simulink model "verify_com_acceleration_computation"  (R2015a)
settings: Solver=ode45  StartTime=0.0  StopTime=1.2  RelTol=1e-3
undefined symbols (not defined in the file or in its folder): A_kalman_transverse, A_kalman_vertical, B_kalman_transverse, B_kalman_vertical, C_kalman_transverse, C_kalman_vertical, com_leg_motor, com_torso, Discrete, g, initial_dx_estimate, initial_dy_estimate, initial_dz_estimate, initial_z_estimate, kalman_stance_slip_threshold, lateral_offset, m_leg, m_leg_motor, m_torso, m_total_real, P0_kalman_transverse, P0_kalman_vertical, pelvis_to_imu, R_kalman_accelerometer, R_kalman_foot_slip, R_kalman_foot_stance, sample_time, Time, X, Y, Z
libraries: nesl_utility x121, sm_lib x43, simulink x3, ctrlSharedLib x3
(part 1 of 3)
settings Model: Creator=wmartin  LastModifiedBy=wmartin

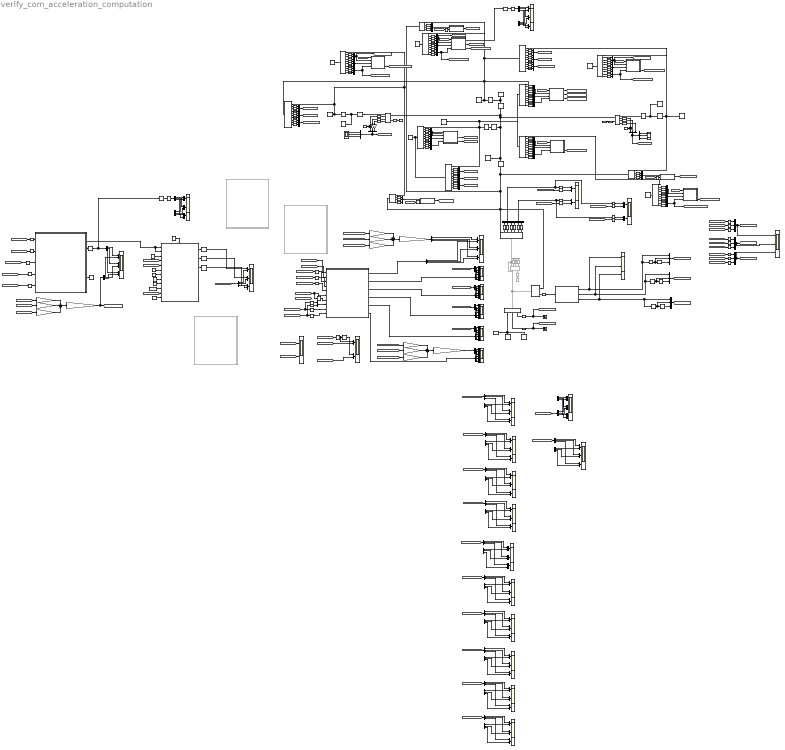
== system verify_com_acceleration_computation ==
  COM Acceleration Yawed Frame : Scope  NumInputPorts=3
      settings: YMin=-0.7~-1.75~-25  YMax=0.7~1.75~5  SaveName=ScopeData29  SampleInput=on
  COM from pelvis : Scope  NumInputPorts=3
      settings: YMin=-0.125~-0.175~-0.15  YMax=0.125~0.2~0.125  SaveName=ScopeData12  SampleInput=on
  Cartesian Joint : sm_lib/Joints/Cartesian Joint  SenseConstraintForce=off  SenseConstraintForceX=off  SenseConstraintForceY=off  SenseConstraintForceZ=off  SenseConstraintTorque=off  SenseConstraintTorqueX=off  SenseConstraintTorqueY=off  SenseConstraintTorqueZ=off  SenseTotalForce=off  SenseTotalForceX=off  SenseTotalForceY=off  SenseTotalForceZ=off  SenseTotalTorque=off  SenseTotalTorqueX=off  SenseTotalTorqueY=off  SenseTotalTorqueZ=off  CompositeWrenchDir=FollowerOnBase  CompositeWrenchFrame=BaseFrame  PxEquilibriumPosition=0  PxEquilibriumPositionUnits=m  PxSpringStiffness=0  PxSpringStiffnessUnits=N/m  PxDampingCoefficient=0  PxDampingCoefficientUnits=N/(m/s)  PxTorqueActuationMode=NoTorque  PxMotionActuationMode=ComputedMotion  PxSensePosition=off  PxSenseVelocity=off  PxSenseAcceleration=off  PxSenseTorqueForce=off  PxPositionTargetSpecify=off  PxPositionTargetPriority=High  PxPositionTargetValue=0  PxPositionTargetValueUnits=m  PxVelocityTargetSpecify=off  PxVelocityTargetPriority=High  PxVelocityTargetValue=0  PxVelocityTargetValueUnits=m/s  PyEquilibriumPosition=0  PyEquilibriumPositionUnits=m  PySpringStiffness=0  PySpringStiffnessUnits=N/m  PyDampingCoefficient=0  PyDampingCoefficientUnits=N/(m/s)  PyTorqueActuationMode=InputTorque  PyMotionActuationMode=ComputedMotion  PySensePosition=off  PySenseVelocity=off  PySenseAcceleration=off  PySenseTorqueForce=off  PyPositionTargetSpecify=off  PyPositionTargetPriority=High  PyPositionTargetValue=0  PyPositionTargetValueUnits=m  PyVelocityTargetSpecify=off  PyVelocityTargetPriority=High  PyVelocityTargetValue=0  PyVelocityTargetValueUnits=m/s  PzEquilibriumPosition=0  PzEquilibriumPositionUnits=m  PzSpringStiffness=0  PzSpringStiffnessUnits=N/m  PzDampingCoefficient=0  PzDampingCoefficientUnits=N/(m/s)  PzTorqueActuationMode=InputTorque  PzMotionActuationMode=ComputedMotion  PzSensePosition=off  PzSenseVelocity=off  PzSenseAcceleration=off  PzSenseTorqueForce=off  PzPositionTargetSpecify=off  PzPositionTargetPriority=High  PzPositionTargetValue=0  PzPositionTargetValueUnits=m  PzVelocityTargetSpecify=off  PzVelocityTargetPriority=High  PzVelocityTargetValue=0  PzVelocityTargetValueUnits=m/s  BlockFunction=simmechanics.library.joints.cartesian_joint
  Compute COM Translational Acceleration (IMU uses non-rotating measurement frame) : MATLAB Function  TreatAsAtomicUnit=on
  Compute COM Translational Acceleration (IMU uses non-rotating measurement frame) (yawed frame as rotated world frame - non rotating) : MATLAB Function  Commented=on  TreatAsAtomicUnit=on
  Compute COM Translational Acceleration (IMU uses rotating measurement frame)1 : MATLAB Function  Commented=on  TreatAsAtomicUnit=on
  Compute COM Translational Acceleration (IMU uses non-rotating measurement frame) : MATLAB Function  Commented=on  TreatAsAtomicUnit=on
  Constant{,1..2,11} (4 alike) : Constant  Value=0
  Constant10 : Constant  Value=true
  Constant12 : Constant  Value=false
  Constant3 : Constant  Value=pi/2
  Constant4 : Constant  Value=pi/2
  Constant5 : Constant  Commented=on  Value=0
  Constant6 : Constant  Value=1000
  Constant7 : Constant  Value=[0 0 0]
  Constant8 : Constant  Value=[0 0 0]
  Constant9 : Constant  Value=[0.1 0 0]
  Demux{,1..42,44..45} (45 alike) : Demux  Outputs=3
  Derivative{,1..12} (13 alike) : Derivative
  Gain{,1,6..7,10..11} (6 alike) : Gain  Gain=m_leg_motor+m_leg
  Gain12 : Gain  Gain=m_torso
  Gain13 : Gain  Gain=1/(m_torso+2*(m_leg_motor+m_leg))
  Gain2 : Gain  Gain=m_torso
  Gain3 : Gain  Gain=1/(m_torso+2*(m_leg_motor+m_leg))
  Gain4 : Gain  Gain=-1
  Gain5 : Gain  Gain=-1
  Gain8 : Gain  Gain=m_torso
  Gain9 : Gain  Gain=1/(m_torso+2*(m_leg_motor+m_leg))
  IMU : sm_lib/Body Elements/Graphic  GraphicType=Marker  MarkerShape=Sphere  MarkerSize=10  MarkerSizeUnits=m  GraphicVisPropType=SimpleVisualProperties  GraphicDiffuseColor=[0.0 0.8 0.8]  GraphicSpecularColor=[0.5 0.5 0.5 1.0]  GraphicAmbientColor=[0.15 0.15 0.15 1.0]  GraphicEmissiveColor=[0.0 0.0 0.0 1.0]  GraphicShininess=75  GraphicOpacity=1.0  BlockFunction=simmechanics.library.body_elements.graphic
  IMU Acceleration Yawed : Scope  NumInputPorts=3
      settings: YMin=-0.3~-1.5~-10  YMax=0.45~6~7  SaveName=ScopeData9  SampleInput=on
  IMU Velocity Yawed : Scope  NumInputPorts=3
      settings: YMin=-0.45~-0.25~-15  YMax=0.2~4~1  SaveName=ScopeData11  SampleInput=on
  Imu to Torso COM yawed : Scope  NumInputPorts=3
      settings: YMin=-0.1175~0.12~-0.2  YMax=-0.095~0.23~0.15  SaveName=ScopeData10  SampleInput=on
  Kalman Filter : Scope  NumInputPorts=3
      settings: YMin=-1000~-1500~-25  YMax=1500~750~35  SaveName=ScopeData23  SampleInput=on
  Kalman Filtering : Subsystem
  L Hip Graphic : sm_lib/Body Elements/Graphic  GraphicType=Marker  MarkerShape=Sphere  MarkerSize=10  MarkerSizeUnits=m  GraphicVisPropType=SimpleVisualProperties  GraphicDiffuseColor=[0.0 0.2 1.0]  GraphicSpecularColor=[0.5 0.5 0.5 1.0]  GraphicAmbientColor=[0.15 0.15 0.15 1.0]  GraphicEmissiveColor=[0.0 0.0 0.0 1.0]  GraphicShininess=75  GraphicOpacity=1.0  BlockFunction=simmechanics.library.body_elements.graphic
  L Hip Yawed : Scope  NumInputPorts=3
      settings: YMin=0.95~0.95~-5  YMax=1.05~1.05~5  SaveName=ScopeData8  SampleInput=on
  LHip  body frame : Scope  NumInputPorts=3
      settings: YMin=0.95~0.95~-5  YMax=1.05~1.05~5  SaveName=ScopeData21  SampleInput=on
  Left Hip Acceleration World Frame : Scope  NumInputPorts=3
      settings: YMin=-0.3~-10~-27.5  YMax=0.9~12.5~7.5  SaveName=ScopeData28  SampleInput=on
  Left Hip Angular Positions / Velocities / Accelerations : Scope  NumInputPorts=3
      settings: YMin=0.95~0.95~-5  YMax=1.05~1.05~5  SaveName=ScopeData2  SampleInput=on
  Left Hip Joint : sm_lib/Joints/Revolute Joint  SenseConstraintForce=off  SenseConstraintForceX=off  SenseConstraintForceY=off  SenseConstraintForceZ=off  SenseConstraintTorque=off  SenseConstraintTorqueX=off  SenseConstraintTorqueY=off  SenseConstraintTorqueZ=off  SenseTotalForce=off  SenseTotalForceX=off  SenseTotalForceY=off  SenseTotalForceZ=off  SenseTotalTorque=off  SenseTotalTorqueX=off  SenseTotalTorqueY=off  SenseTotalTorqueZ=off  CompositeWrenchDir=FollowerOnBase  CompositeWrenchFrame=BaseFrame  EquilibriumPosition=0  EquilibriumPositionUnits=deg  SpringStiffness=0  SpringStiffnessUnits=N*m/deg  DampingCoefficient=0  DampingCoefficientUnits=N*m/(deg/s)  TorqueActuationMode=InputTorque  MotionActuationMode=ComputedMotion  SensePosition=on  SenseVelocity=on  SenseAcceleration=on  SenseTorqueForce=off  PositionTargetSpecify=off  PositionTargetPriority=High  PositionTargetValue=0  PositionTargetValueUnits=deg  VelocityTargetSpecify=off  VelocityTargetPriority=High  VelocityTargetValue=0  VelocityTargetValueUnits=deg/s  BlockFunction=simmechanics.library.joints.revolute_joint
  Left Hip Mass : sm_lib/Body Elements/Solid  InertiaType=Custom  Mass=m_leg_motor+m_leg  MassUnits=kg  CenterOfMass=com_leg_motor  CenterOfMassUnits=m  MomentsOfInertia=[1 1 1]  MomentsOfInertiaUnits=kg*m^2  ProductsOfInertia=[0 0 0]  ProductsOfInertiaUnits=kg*m^2  DensityBased=on  Density=1000  DensityUnits=kg/(m^3)  GraphicType=None  MarkerShape=Sphere  MarkerSize=10  MarkerSizeUnits=m  GraphicVisPropType=SimpleVisualProperties  GraphicDiffuseColor=[0.5 0.5 0.5]  GraphicSpecularColor=[0.5 0.5 0.5 1.0]  GraphicAmbientColor=[0.15 0.15 0.15 1.0]  GraphicEmissiveColor=[0.0 0.0 0.0 1.0]  GraphicShininess=75  GraphicOpacity=1.0  GeometryShape=Sphere  RectangleSize=[1 1]  RectangleSizeUnits=m  BrickDimensions=[1 1 1]  BrickDimensionUnits=m  CylinderRadius=1  CylinderRadiusUnits=m  CylinderLength=1  CylinderLengthUnits=m  SphereRadius=0.15  SphereRadiusUnits=m  EllipsoidRadii=[1 1 1]  EllipsoidRadiiUnits=m  ExtrusionCrossSection=[1 1; -1 1; -1 -1; 1 -1]  ExtrusionCrossSectionUnits=m  ExtrusionLength=1  ExtrusionLengthUnits=m  PolygonNumSides=3  PolygonOuterRadius=1  PolygonOuterRadiusUnits=m  ExtGeomFileType=STL  ExtGeomFileUnits=m  RevolutionCrossSection=[1 1; 1 -1; 2 -1; 2 1]  RevolutionCrossSectionUnits=m  RevolutionExtent=Full  RevolutionAngle=180  RevolutionAngleUnits=deg  BlockFunction=simmechanics.library.body_elements.solid
  Mechanism Configuration : sm_lib/Utilities/Mechanism Configuration  UniformGravity=Constant  GravityVector=[0 0 -9.80665]  GravityUnits=m/s^2  LinearizationDelta=0.001  BlockFunction=simmechanics.library.utilities.mechanism_configuration
  Mux{1..4,10..12,26..27,32..36,38,45..50,52,57,61..63,67..68,73..81,85..87,91..93} (43 alike) : Mux  Inputs=3
  Mux{5..9,13..25,28..31,37,39..41,43..44,51,53..56,58..60,64..66,69..72,82..84,88..90,94..117} (73 alike) : Mux  Inputs=2
  Mux42 : Mux  Commented=on  Inputs=3
  PS-Simulink Converter{,1..42,46..114} (112 alike) : nesl_utility/PS-Simulink Converter  PhysicalDomain=network_engine_domain  SubClassName=ps_output  LeftPortType=input  RightPortType=output  PseudoPeriodic=off  Frequencies=[]  Unit=1  AffineConversion=off
  PS-Simulink Converter43 : nesl_utility/PS-Simulink Converter  Commented=on  PhysicalDomain=network_engine_domain  SubClassName=ps_output  LeftPortType=input  RightPortType=output  PseudoPeriodic=off  Frequencies=[]  Unit=1  AffineConversion=off
  PS-Simulink Converter44 : nesl_utility/PS-Simulink Converter  Commented=on  PhysicalDomain=network_engine_domain  SubClassName=ps_output  LeftPortType=input  RightPortType=output  PseudoPeriodic=off  Frequencies=[]  Unit=1  AffineConversion=off
  PS-Simulink Converter45 : nesl_utility/PS-Simulink Converter  Commented=on  PhysicalDomain=network_engine_domain  SubClassName=ps_output  LeftPortType=input  RightPortType=output  PseudoPeriodic=off  Frequencies=[]  Unit=1  AffineConversion=off
  Pelvic Rotation to World{,1..3} (4 alike) : sm_lib/Frames and Transforms/Rigid Transform  TranslationMethod=None  TranslationLengthUnit=m  TranslationStandardAxis=+Z  TranslationStandardOffset=0  TranslationCartesianOffset=[0 0 0]  TranslationROffset=0  TranslationROffsetUnits=m  TranslationZOffset=0  TranslationZOffsetUnits=m  TranslationThetaOffset=0  TranslationThetaOffsetUnits=deg  RotationMethod=AlignedAxes  RotationAngleUnits=deg  RotationStandardAxis=+Z  RotationAngle=0.0  RotationArbitraryAxis=[0 0 1]  FollAlignAxisA=+X  BaseAlignAxisA=+Z  FollAlignAxisB=+Y  BaseAlignAxisB=+Y  RotationMatrix=[1 0 0; 0 1 0; 0 0 1]  BlockFunction=simmechanics.library.frames_transforms.rigid_transform
  Pelvis : sm_lib/Body Elements/Graphic  GraphicType=Marker  MarkerShape=Sphere  MarkerSize=10  MarkerSizeUnits=m  GraphicVisPropType=SimpleVisualProperties  GraphicDiffuseColor=[1.0 0.0 1.0]  GraphicSpecularColor=[0.5 0.5 0.5 1.0]  GraphicAmbientColor=[0.15 0.15 0.15 1.0]  GraphicEmissiveColor=[0.0 0.0 0.0 1.0]  GraphicShininess=75  GraphicOpacity=1.0  BlockFunction=simmechanics.library.body_elements.graphic
  Pelvis Acceleration World Frame : Scope  NumInputPorts=3
      settings: YMin=-0.5~-2.5~-17.5  YMax=1~4~7.5  SaveName=ScopeData26  SampleInput=on
  Pelvis Acceleration from Ground Yawed : Scope  NumInputPorts=3
      settings: YMin=0.95~0.95~-5  YMax=1.05~1.05~5  SaveName=ScopeData19  SampleInput=on
  Pelvis Acceleration from IMU Yawed : Scope  NumInputPorts=3
      settings: YMin=0.95~0.95~-5  YMax=1.05~1.05~5  SaveName=ScopeData18  SampleInput=on
  Pelvis to COM Accleration Yawed : Scope  NumInputPorts=3
      settings: YMin=-9~-15~-25  YMax=8~20~25  SaveName=ScopeData25  SampleInput=on
  Pelvis to IMU : sm_lib/Frames and Transforms/Rigid Transform  TranslationMethod=Cartesian  TranslationLengthUnit=m  TranslationStandardAxis=+Z  TranslationStandardOffset=0  TranslationCartesianOffset=pelvis_to_imu  TranslationROffset=0  TranslationROffsetUnits=m  TranslationZOffset=0  TranslationZOffsetUnits=m  TranslationThetaOffset=0  TranslationThetaOffsetUnits=deg  RotationMethod=None  RotationAngleUnits=deg  RotationStandardAxis=+Z  RotationAngle=0.0  RotationArbitraryAxis=[0 0 1]  FollAlignAxisA=+X  BaseAlignAxisA=+Y  FollAlignAxisB=+Y  BaseAlignAxisB=+Z  RotationMatrix=[1 0 0; 0 1 0; 0 0 1]  BlockFunction=simmechanics.library.frames_transforms.rigid_transform
  Pelvis to L Hip COM : sm_lib/Frames and Transforms/Rigid Transform  TranslationMethod=Cartesian  TranslationLengthUnit=m  TranslationStandardAxis=+Z  TranslationStandardOffset=0  TranslationCartesianOffset=com_leg_motor  TranslationROffset=0  TranslationROffsetUnits=m  TranslationZOffset=0  TranslationZOffsetUnits=m  TranslationThetaOffset=0  TranslationThetaOffsetUnits=deg  RotationMethod=None  RotationAngleUnits=deg  RotationStandardAxis=+Z  RotationAngle=-90  RotationArbitraryAxis=[0 0 1]  FollAlignAxisA=+Z  BaseAlignAxisA=+X  FollAlignAxisB=+Y  BaseAlignAxisB=+Y  RotationMatrix=[1 0 0; 0 1 0; 0 0 1]  BlockFunction=simmechanics.library.frames_transforms.rigid_transform
  Pelvis to R Hip COM : sm_lib/Frames and Transforms/Rigid Transform  TranslationMethod=Cartesian  TranslationLengthUnit=m  TranslationStandardAxis=+Z  TranslationStandardOffset=0  TranslationCartesianOffset=com_leg_motor.*[1,-1,1]  TranslationROffset=0  TranslationROffsetUnits=m  TranslationZOffset=0  TranslationZOffsetUnits=m  TranslationThetaOffset=0  TranslationThetaOffsetUnits=deg  RotationMethod=None  RotationAngleUnits=deg  RotationStandardAxis=+Z  RotationAngle=-90  RotationArbitraryAxis=[0 0 1]  FollAlignAxisA=+Z  BaseAlignAxisA=+X  FollAlignAxisB=+Y  BaseAlignAxisB=+Y  RotationMatrix=[1 0 0; 0 1 0; 0 0 1]  BlockFunction=simmechanics.library.frames_transforms.rigid_transform
  Pelvis to Trunk COM : sm_lib/Frames and Transforms/Rigid Transform  TranslationMethod=Cartesian  TranslationLengthUnit=m  TranslationStandardAxis=+Z  TranslationStandardOffset=0  TranslationCartesianOffset=com_torso  TranslationROffset=0  TranslationROffsetUnits=m  TranslationZOffset=0  TranslationZOffsetUnits=m  TranslationThetaOffset=0  TranslationThetaOffsetUnits=deg  RotationMethod=None  RotationAngleUnits=deg  RotationStandardAxis=+Z  RotationAngle=-90  RotationArbitraryAxis=[0 0 1]  FollAlignAxisA=+Z  BaseAlignAxisA=+X  FollAlignAxisB=+Y  BaseAlignAxisB=+Y  RotationMatrix=[1 0 0; 0 1 0; 0 0 1]  BlockFunction=simmechanics.library.frames_transforms.rigid_transform
  PositionUsingRobotGeometry : MATLAB Function  TreatAsAtomicUnit=on
  R Hip Graphic : sm_lib/Body Elements/Graphic  GraphicType=Marker  MarkerShape=Sphere  MarkerSize=10  MarkerSizeUnits=m  GraphicVisPropType=SimpleVisualProperties  GraphicDiffuseColor=[1.0 0.0 0.2]  GraphicSpecularColor=[0.5 0.5 0.5 1.0]  GraphicAmbientColor=[0.15 0.15 0.15 1.0]  GraphicEmissiveColor=[0.0 0.0 0.0 1.0]  GraphicShininess=75  GraphicOpacity=1.0  BlockFunction=simmechanics.library.body_elements.graphic
  R Hip Yawed : Scope  NumInputPorts=3
      settings: YMin=0.95~0.95~-5  YMax=1.05~1.05~5  SaveName=ScopeData4  SampleInput=on
  RHip  body frame : Scope  NumInputPorts=3
      settings: YMin=-1e-15~-1.5~-1  YMax=1e-15~1.5~1.3  SaveName=ScopeData20  SampleInput=on
  Right Hip Acceleration World Frame : Scope  NumInputPorts=3
      settings: YMin=-0.3~-10~-27.5  YMax=0.9~12.5~7.5  SaveName=ScopeData27  SampleInput=on
  Right Hip Angular Positions / Velocities / Accelerations : Scope  NumInputPorts=3
      settings: YMin=0.95~0.95~-5  YMax=1.05~1.05~5  SampleInput=on
  Right Hip Joint : sm_lib/Joints/Revolute Joint  SenseConstraintForce=off  SenseConstraintForceX=off  SenseConstraintForceY=off  SenseConstraintForceZ=off  SenseConstraintTorque=off  SenseConstraintTorqueX=off  SenseConstraintTorqueY=off  SenseConstraintTorqueZ=off  SenseTotalForce=off  SenseTotalForceX=off  SenseTotalForceY=off  SenseTotalForceZ=off  SenseTotalTorque=off  SenseTotalTorqueX=off  SenseTotalTorqueY=off  SenseTotalTorqueZ=off  CompositeWrenchDir=FollowerOnBase  CompositeWrenchFrame=BaseFrame  EquilibriumPosition=0  EquilibriumPositionUnits=deg  SpringStiffness=0  SpringStiffnessUnits=N*m/deg  DampingCoefficient=0  DampingCoefficientUnits=N*m/(deg/s)  TorqueActuationMode=InputTorque  MotionActuationMode=ComputedMotion  SensePosition=on  SenseVelocity=on  SenseAcceleration=on  SenseTorqueForce=off  PositionTargetSpecify=on  PositionTargetPriority=High  PositionTargetValue=0  PositionTargetValueUnits=deg  VelocityTargetSpecify=off  VelocityTargetPriority=High  VelocityTargetValue=0  VelocityTargetValueUnits=deg/s  BlockFunction=simmechanics.library.joints.revolute_joint
  Right Hip Mass : sm_lib/Body Elements/Solid  InertiaType=Custom  Mass=m_leg_motor+m_leg  MassUnits=kg  CenterOfMass=com_leg_motor.*[1,-1,1]  CenterOfMassUnits=m  MomentsOfInertia=[1 1 1]  MomentsOfInertiaUnits=kg*m^2  ProductsOfInertia=[0 0 0]  ProductsOfInertiaUnits=kg*m^2  DensityBased=on  Density=1000  DensityUnits=kg/(m^3)  GraphicType=None  MarkerShape=Sphere  MarkerSize=10  MarkerSizeUnits=m  GraphicVisPropType=SimpleVisualProperties  GraphicDiffuseColor=[0.5 0.5 0.5]  GraphicSpecularColor=[0.5 0.5 0.5 1.0]  GraphicAmbientColor=[0.15 0.15 0.15 1.0]  GraphicEmissiveColor=[0.0 0.0 0.0 1.0]  GraphicShininess=75  GraphicOpacity=1.0  GeometryShape=Sphere  RectangleSize=[1 1]  RectangleSizeUnits=m  BrickDimensions=[1 1 1]  BrickDimensionUnits=m  CylinderRadius=1  CylinderRadiusUnits=m  CylinderLength=1  CylinderLengthUnits=m  SphereRadius=0.15  SphereRadiusUnits=m  EllipsoidRadii=[1 1 1]  EllipsoidRadiiUnits=m  ExtrusionCrossSection=[1 1; -1 1; -1 -1; 1 -1]  ExtrusionCrossSectionUnits=m  ExtrusionLength=1  ExtrusionLengthUnits=m  PolygonNumSides=3  PolygonOuterRadius=1  PolygonOuterRadiusUnits=m  ExtGeomFileType=STL  ExtGeomFileUnits=m  RevolutionCrossSection=[1 1; 1 -1; 2 -1; 2 1]  RevolutionCrossSectionUnits=m  RevolutionExtent=Full  RevolutionAngle=180  RevolutionAngleUnits=deg  BlockFunction=simmechanics.library.body_elements.solid
  Right and Left Hip Angles : Scope  NumInputPorts=2
      settings: YMin=0.95~0.95  YMax=1.05~1.05  SaveName=ScopeData14  SampleInput=on
  Roll and Pitch Joint : sm_lib/Joints/Universal Joint  SenseConstraintForce=off  SenseConstraintForceX=off  SenseConstraintForceY=off  SenseConstraintForceZ=off  SenseConstraintTorque=off  SenseConstraintTorqueX=off  SenseConstraintTorqueY=off  SenseConstraintTorqueZ=off  SenseTotalForce=off  SenseTotalForceX=off  SenseTotalForceY=off  SenseTotalForceZ=off  SenseTotalTorque=off  SenseTotalTorqueX=off  SenseTotalTorqueY=off  SenseTotalTorqueZ=off  CompositeWrenchDir=FollowerOnBase  CompositeWrenchFrame=BaseFrame  RxEquilibriumPosition=0  RxEquilibriumPositionUnits=deg  RxSpringStiffness=0  RxSpringStiffnessUnits=N*m/deg  RxDampingCoefficient=0  RxDampingCoefficientUnits=N*m/(deg/s)  RxTorqueActuationMode=NoTorque  RxMotionActuationMode=ComputedMotion  RxSensePosition=on  RxSenseVelocity=on  RxSenseAcceleration=on  RxSenseTorqueForce=off  RxPositionTargetSpecify=off  RxPositionTargetPriority=High  RxPositionTargetValue=20  RxPositionTargetValueUnits=deg  RxVelocityTargetSpecify=off  RxVelocityTargetPriority=High  RxVelocityTargetValue=0  RxVelocityTargetValueUnits=deg/s  RyEquilibriumPosition=0  RyEquilibriumPositionUnits=deg  RySpringStiffness=0  RySpringStiffnessUnits=N*m/deg  RyDampingCoefficient=0  RyDampingCoefficientUnits=N*m/(deg/s)  RyTorqueActuationMode=NoTorque  RyMotionActuationMode=ComputedMotion  RySensePosition=on  RySenseVelocity=on  RySenseAcceleration=on  RySenseTorqueForce=off  RyPositionTargetSpecify=off  RyPositionTargetPriority=High  RyPositionTargetValue=0  RyPositionTargetValueUnits=deg  RyVelocityTargetSpecify=off  RyVelocityTargetPriority=High  RyVelocityTargetValue=0  RyVelocityTargetValueUnits=deg/s  BlockFunction=simmechanics.library.joints.universal_joint
  Rotate to from World to Yawed Frame1 : MATLAB Function  TreatAsAtomicUnit=on
  Rotate to from World to Yawed Frame2 : MATLAB Function  TreatAsAtomicUnit=on
  Rotate to from World to Yawed Frame3 : MATLAB Function  TreatAsAtomicUnit=on
  Rotation To Euler Angles : MATLAB Function  TreatAsAtomicUnit=on
  Selector{,1,4..7,14..15,26,33} (10 alike) : Selector  InputPortWidth=3  Indices=[1 2]
  Selector{10..11,22..25,31} (7 alike) : Selector  InputPortWidth=3  Indices=[2]
  Selector{2..3,12..13,29,34..36} (8 alike) : Selector  InputPortWidth=3  Indices=[3]
  Selector16 : Selector  InputPortWidth=9  Indices=[4 5 6]
  Selector{8..9,17..20,27..28,30,32} (10 alike) : Selector  InputPortWidth=3  Indices=[1]
  Selector21 : Selector  InputPortWidth=9  Indices=[4 5 6]
  Simulink-PS Converter : nesl_utility/Simulink-PS Converter  PhysicalDomain=network_engine_domain  SubClassName=ps_input  LeftPortType=input  RightPortType=output  PseudoPeriodic=off  Frequencies=[]  NoiseDistribution=none  NoiseParameters=[]  Unit=1  AffineConversion=off  InputFiltering=off  SimscapeFilterOrder=1  InputFilterTimeConstant=0.001  UdotUserProvided=1
  Simulink-PS Converter1 : nesl_utility/Simulink-PS Converter  PhysicalDomain=network_engine_domain  SubClassName=ps_input  LeftPortType=input  RightPortType=output  PseudoPeriodic=off  Frequencies=[]  NoiseDistribution=none  NoiseParameters=[]  Unit=1  AffineConversion=off  InputFiltering=off  SimscapeFilterOrder=1  InputFilterTimeConstant=0.001  UdotUserProvided=1
  Simulink-PS Converter2 : nesl_utility/Simulink-PS Converter  Commented=on  PhysicalDomain=network_engine_domain  SubClassName=ps_input  LeftPortType=input  RightPortType=output  PseudoPeriodic=off  Frequencies=[]  NoiseDistribution=none  NoiseParameters=[]  Unit=1  AffineConversion=off  InputFiltering=off  SimscapeFilterOrder=1  InputFilterTimeConstant=0.001  UdotUserProvided=1
  Simulink-PS Converter3 : nesl_utility/Simulink-PS Converter  PhysicalDomain=network_engine_domain  SubClassName=ps_input  LeftPortType=input  RightPortType=output  PseudoPeriodic=off  Frequencies=[]  NoiseDistribution=none  NoiseParameters=[]  Unit=1  AffineConversion=off  InputFiltering=on  SimscapeFilterOrder=2  InputFilterTimeConstant=0.001  UdotUserProvided=1
  Simulink-PS Converter4 : nesl_utility/Simulink-PS Converter  PhysicalDomain=network_engine_domain  SubClassName=ps_input  LeftPortType=input  RightPortType=output  PseudoPeriodic=off  Frequencies=[]  NoiseDistribution=none  NoiseParameters=[]  Unit=1  AffineConversion=off  InputFiltering=on  SimscapeFilterOrder=2  InputFilterTimeConstant=0.001  UdotUserProvided=1
  Sine Wave : Sin  Amplitude=900  Frequency=5  SampleTime=0
  Sine Wave1 : Sin  Amplitude=100  Frequency=5  SampleTime=0
  Solver Configuration : nesl_utility/Solver Configuration  PhysicalDomain=network_engine_domain  SubClassName=solver  LeftPortType=input  RightPortType=generic  Accelerate=off  Tones=[]  Harmonics=[]  SimulateNoise=off  Profile=off  UseLocalSampling=off  EnableSwitchedLinearOptims=on  FrequencyDomain=off  UseCCode=off  RelTol=0.001  AbsTol=1e-06  MinStep=1e-09  ToWorkspace=off  RevertToSquareIcSolve=off  NumHomotopyIterations=100  DoDC=off  ResidualTolerance=1e-09  UseLocalSolver=off  LocalSolverChoice=NE_BACKWARD_EULER_ADVANCER  LocalSolverSampleTime=0.001  DoFixedCost=off  MaxNonlinIter=3  MaxModeIter=2  LinearAlgebra=Sparse  DelaysMemoryBudget=1024  AutomaticFiltering=on  FilteringTimeConstant=0.001
  Sum : Sum  Inputs=+++
  Sum1 : Sum  Inputs=+-|
  Sum2 : Sum  Inputs=++|
  Sum3 : Sum  Inputs=+++
  Sum4 : Sum  Inputs=+++
  System COM Acceleration World Frame : Scope  NumInputPorts=3
      settings: YMin=-0.07~-1.75~-25  YMax=0.005~1.75~5  SaveName=ScopeData3  SampleInput=on
  Torso COM Acceleration World Frame : Scope  NumInputPorts=3
      settings: YMin=-0.0075~-18~-42.5  YMax=0.0175~4~7.5  SaveName=ScopeData5  SampleInput=on
  Torso COM Acceleration Relative to IMU : Scope  NumInputPorts=3
      settings: YMin=-1~-20~-15  YMax=2.25~5~17.5  SaveName=ScopeData6  SampleInput=on
  Torso COM Velocity Relative to IMU : Scope  NumInputPorts=3
      settings: YMin=-0.045~-0.25~0  YMax=0~0.35~0.8  SaveName=ScopeData7  SampleInput=on
  Torso COM Yawed Accel : Scope  NumInputPorts=3
      settings: YMin=-7~-30~-35  YMax=7~30~40  SaveName=ScopeData24  SampleInput=on
  Torso Graphic : sm_lib/Body Elements/Graphic  GraphicType=Marker  MarkerShape=Sphere  MarkerSize=10  MarkerSizeUnits=m  GraphicVisPropType=SimpleVisualProperties  GraphicDiffuseColor=[0.2 0.8 0.0]  GraphicSpecularColor=[0.5 0.5 0.5 1.0]  GraphicAmbientColor=[0.15 0.15 0.15 1.0]  GraphicEmissiveColor=[0.0 0.0 0.0 1.0]  GraphicShininess=75  GraphicOpacity=1.0  BlockFunction=simmechanics.library.body_elements.graphic
  "Torso Position, Velocity, Acceleration" : Scope  NumInputPorts=3
      settings: YMin=0.95~0.95~-5  YMax=1.05~1.05~5  SaveName=ScopeData13  SampleInput=on
  Torso Roll Pitch Comparison Position : Scope  NumInputPorts=2
      settings: YMin=0.95~0.95  YMax=1.05~1.05  SaveName=ScopeData15  SampleInput=on
  Torso Roll Pitch Comparison Velocity : Scope  NumInputPorts=2
      settings: YMin=0.95~0.95  YMax=1.05~1.05  SaveName=ScopeData17  SampleInput=on
  Torso Velocity Yawed : Scope  NumInputPorts=3
      settings: YMin=-0.09~-0.1~-13  YMax=0.1~1.9~1  SaveName=ScopeData22  SampleInput=on
  Transform Sensor : sm_lib/Frames and Transforms/Transform Sensor  MeasurementFrame=World  SenseAngle=off  SenseAxis=off  SenseAngle1=off  SenseAngle2=off  SenseAngle3=off  SenseQ=off  SenseR=on  SenseOmegaX=off  SenseOmegaY=off  SenseOmegaZ=off  SenseOmega1=off  SenseOmega2=off  SenseOmega3=off  SenseQDot=off  SenseRDot=off  SenseAlphaX=off  SenseAlphaY=off  SenseAlphaZ=off  SenseAlpha1=off  SenseAlpha2=off  SenseAlpha3=off  SenseQDDot=off  SenseRDDot=off  SenseX=off  SenseY=off  SenseZ=off  SenseRad=off  SenseAzim=off  SenseDist=off  SenseInc=off  SenseXDot=off  SenseYDot=off  SenseZDot=off  SenseRadDot=off  SenseAzimDot=off  SenseDistDot=off  SenseIncDot=off  SenseXDDot=off  SenseYDDot=off  SenseZDDot=off  SenseRadDDot=off  SenseAzimDDot=off  SenseDistDDot=off  SenseIncDDot=off  BlockFunction=simmechanics.library.frames_transforms.transform_sensor
  Transform Sensor{1,3..5,12..13} (6 alike) : sm_lib/Frames and Transforms/Transform Sensor  MeasurementFrame=World  SenseAngle=off  SenseAxis=off  SenseAngle1=off  SenseAngle2=off  SenseAngle3=off  SenseQ=off  SenseR=off  SenseOmegaX=off  SenseOmegaY=off  SenseOmegaZ=off  SenseOmega1=off  SenseOmega2=off  SenseOmega3=off  SenseQDot=off  SenseRDot=off  SenseAlphaX=off  SenseAlphaY=off  SenseAlphaZ=off  SenseAlpha1=off  SenseAlpha2=off  SenseAlpha3=off  SenseQDDot=off  SenseRDDot=off  SenseX=on  SenseY=on  SenseZ=on  SenseRad=off  SenseAzim=off  SenseDist=off  SenseInc=off  SenseXDot=on  SenseYDot=on  SenseZDot=on  SenseRadDot=off  SenseAzimDot=off  SenseDistDot=off  SenseIncDot=off  SenseXDDot=on  SenseYDDot=on  SenseZDDot=on  SenseRadDDot=off  SenseAzimDDot=off  SenseDistDDot=off  SenseIncDDot=off  BlockFunction=simmechanics.library.frames_transforms.transform_sensor
  Transform Sensor10 : sm_lib/Frames and Transforms/Transform Sensor  MeasurementFrame=World  SenseAngle=off  SenseAxis=off  SenseAngle1=off  SenseAngle2=off  SenseAngle3=off  SenseQ=off  SenseR=off  SenseOmegaX=off  SenseOmegaY=off  SenseOmegaZ=off  SenseOmega1=off  SenseOmega2=off  SenseOmega3=off  SenseQDot=off  SenseRDot=off  SenseAlphaX=off  SenseAlphaY=off  SenseAlphaZ=off  SenseAlpha1=off  SenseAlpha2=off  SenseAlpha3=off  SenseQDDot=off  SenseRDDot=off  SenseX=on  SenseY=on  SenseZ=on  SenseRad=off  SenseAzim=off  SenseDist=off  SenseInc=off  SenseXDot=off  SenseYDot=off  SenseZDot=off  SenseRadDot=off  SenseAzimDot=off  SenseDistDot=off  SenseIncDot=off  SenseXDDot=off  SenseYDDot=off  SenseZDDot=off  SenseRadDDot=off  SenseAzimDDot=off  SenseDistDDot=off  SenseIncDDot=off  BlockFunction=simmechanics.library.frames_transforms.transform_sensor
  Transform Sensor11 : sm_lib/Frames and Transforms/Transform Sensor  MeasurementFrame=World  SenseAngle=off  SenseAxis=off  SenseAngle1=off  SenseAngle2=off  SenseAngle3=off  SenseQ=off  SenseR=off  SenseOmegaX=off  SenseOmegaY=off  SenseOmegaZ=off  SenseOmega1=off  SenseOmega2=off  SenseOmega3=off  SenseQDot=off  SenseRDot=off  SenseAlphaX=off  SenseAlphaY=off  SenseAlphaZ=off  SenseAlpha1=off  SenseAlpha2=off  SenseAlpha3=off  SenseQDDot=off  SenseRDDot=off  SenseX=on  SenseY=on  SenseZ=on  SenseRad=off  SenseAzim=off  SenseDist=off  SenseInc=off  SenseXDot=off  SenseYDot=off  SenseZDot=off  SenseRadDot=off  SenseAzimDot=off  SenseDistDot=off  SenseIncDot=off  SenseXDDot=off  SenseYDDot=off  SenseZDDot=off  SenseRadDDot=off  SenseAzimDDot=off  SenseDistDDot=off  SenseIncDDot=off  BlockFunction=simmechanics.library.frames_transforms.transform_sensor
  Transform Sensor2 : sm_lib/Frames and Transforms/Transform Sensor  MeasurementFrame=Base  SenseAngle=off  SenseAxis=off  SenseAngle1=off  SenseAngle2=off  SenseAngle3=off  SenseQ=off  SenseR=off  SenseOmegaX=off  SenseOmegaY=off  SenseOmegaZ=off  SenseOmega1=off  SenseOmega2=off  SenseOmega3=off  SenseQDot=off  SenseRDot=off  SenseAlphaX=off  SenseAlphaY=off  SenseAlphaZ=off  SenseAlpha1=off  SenseAlpha2=off  SenseAlpha3=off  SenseQDDot=off  SenseRDDot=off  SenseX=on  SenseY=on  SenseZ=on  SenseRad=off  SenseAzim=off  SenseDist=off  SenseInc=off  SenseXDot=on  SenseYDot=on  SenseZDot=on  SenseRadDot=off  SenseAzimDot=off  SenseDistDot=off  SenseIncDot=off  SenseXDDot=on  SenseYDDot=on  SenseZDDot=on  SenseRadDDot=off  SenseAzimDDot=off  SenseDistDDot=off  SenseIncDDot=off  BlockFunction=simmechanics.library.frames_transforms.transform_sensor
  Transform Sensor6 : sm_lib/Frames and Transforms/Transform Sensor  MeasurementFrame=NonRotatingFollower  SenseAngle=off  SenseAxis=off  SenseAngle1=off  SenseAngle2=off  SenseAngle3=off  SenseQ=off  SenseR=off  SenseOmegaX=off  SenseOmegaY=off  SenseOmegaZ=off  SenseOmega1=off  SenseOmega2=off  SenseOmega3=off  SenseQDot=off  SenseRDot=off  SenseAlphaX=off  SenseAlphaY=off  SenseAlphaZ=off  SenseAlpha1=off  SenseAlpha2=off  SenseAlpha3=off  SenseQDDot=off  SenseRDDot=off  SenseX=on  SenseY=on  SenseZ=on  SenseRad=off  SenseAzim=off  SenseDist=off  SenseInc=off  SenseXDot=on  SenseYDot=on  SenseZDot=on  SenseRadDot=off  SenseAzimDot=off  SenseDistDot=off  SenseIncDot=off  SenseXDDot=on  SenseYDDot=on  SenseZDDot=on  SenseRadDDot=off  SenseAzimDDot=off  SenseDistDDot=off  SenseIncDDot=off  BlockFunction=simmechanics.library.frames_transforms.transform_sensor
  Transform Sensor7 : sm_lib/Frames and Transforms/Transform Sensor  MeasurementFrame=Base  SenseAngle=off  SenseAxis=off  SenseAngle1=off  SenseAngle2=off  SenseAngle3=off  SenseQ=off  SenseR=off  SenseOmegaX=off  SenseOmegaY=off  SenseOmegaZ=off  SenseOmega1=off  SenseOmega2=off  SenseOmega3=off  SenseQDot=off  SenseRDot=off  SenseAlphaX=off  SenseAlphaY=off  SenseAlphaZ=off  SenseAlpha1=off  SenseAlpha2=off  SenseAlpha3=off  SenseQDDot=off  SenseRDDot=off  SenseX=on  SenseY=on  SenseZ=on  SenseRad=off  SenseAzim=off  SenseDist=off  SenseInc=off  SenseXDot=on  SenseYDot=on  SenseZDot=on  SenseRadDot=off  SenseAzimDot=off  SenseDistDot=off  SenseIncDot=off  SenseXDDot=on  SenseYDDot=on  SenseZDDot=on  SenseRadDDot=off  SenseAzimDDot=off  SenseDistDDot=off  SenseIncDDot=off  BlockFunction=simmechanics.library.frames_transforms.transform_sensor
  Transform Sensor8 : sm_lib/Frames and Transforms/Transform Sensor  MeasurementFrame=Base  SenseAngle=off  SenseAxis=off  SenseAngle1=off  SenseAngle2=off  SenseAngle3=off  SenseQ=off  SenseR=off  SenseOmegaX=off  SenseOmegaY=off  SenseOmegaZ=off  SenseOmega1=off  SenseOmega2=off  SenseOmega3=off  SenseQDot=off  SenseRDot=off  SenseAlphaX=off  SenseAlphaY=off  SenseAlphaZ=off  SenseAlpha1=off  SenseAlpha2=off  SenseAlpha3=off  SenseQDDot=off  SenseRDDot=off  SenseX=on  SenseY=on  SenseZ=on  SenseRad=off  SenseAzim=off  SenseDist=off  SenseInc=off  SenseXDot=on  SenseYDot=on  SenseZDot=on  SenseRadDot=off  SenseAzimDot=off  SenseDistDot=off  SenseIncDot=off  SenseXDDot=on  SenseYDDot=on  SenseZDDot=on  SenseRadDDot=off  SenseAzimDDot=off  SenseDistDDot=off  SenseIncDDot=off  BlockFunction=simmechanics.library.frames_transforms.transform_sensor
  Transform Sensor9 : sm_lib/Frames and Transforms/Transform Sensor  MeasurementFrame=World  SenseAngle=off  SenseAxis=off  SenseAngle1=off  SenseAngle2=off  SenseAngle3=off  SenseQ=off  SenseR=off  SenseOmegaX=off  SenseOmegaY=off  SenseOmegaZ=off  SenseOmega1=off  SenseOmega2=off  SenseOmega3=off  SenseQDot=off  SenseRDot=off  SenseAlphaX=off  SenseAlphaY=off  SenseAlphaZ=off  SenseAlpha1=off  SenseAlpha2=off  SenseAlpha3=off  SenseQDDot=off  SenseRDDot=off  SenseX=on  SenseY=on  SenseZ=on  SenseRad=off  SenseAzim=off  SenseDist=off  SenseInc=off  SenseXDot=off  SenseYDot=off  SenseZDot=off  SenseRadDot=off  SenseAzimDot=off  SenseDistDot=off  SenseIncDot=off  SenseXDDot=off  SenseYDDot=off  SenseZDDot=off  SenseRadDDot=off  SenseAzimDDot=off  SenseDistDDot=off  SenseIncDDot=off  BlockFunction=simmechanics.library.frames_transforms.transform_sensor
  Transform Roll Pitch Yaw : Scope  NumInputPorts=3
      settings: YMin=0~0~-2.25e-16  YMax=1.7~0.275~3e-16  SaveName=ScopeData16  SampleInput=on
  Trunk Mass : sm_lib/Body Elements/Solid  InertiaType=Custom  Mass=m_torso  MassUnits=kg  CenterOfMass=com_torso  CenterOfMassUnits=m  MomentsOfInertia=[1 1 1]  MomentsOfInertiaUnits=kg*m^2  ProductsOfInertia=[0 0 0]  ProductsOfInertiaUnits=kg*m^2  DensityBased=on  Density=1000  DensityUnits=kg/(m^3)  GraphicType=None  MarkerShape=Sphere  MarkerSize=10  MarkerSizeUnits=m  GraphicVisPropType=SimpleVisualProperties  GraphicDiffuseColor=[0.5 0.5 0.5]  GraphicSpecularColor=[0.5 0.5 0.5 1.0]  GraphicAmbientColor=[0.15 0.15 0.15 1.0]  GraphicEmissiveColor=[0.0 0.0 0.0 1.0]  GraphicShininess=75  GraphicOpacity=1.0  GeometryShape=Sphere  RectangleSize=[1 1]  RectangleSizeUnits=m  BrickDimensions=[1 1 1]  BrickDimensionUnits=m  CylinderRadius=1  CylinderRadiusUnits=m  CylinderLength=1  CylinderLengthUnits=m  SphereRadius=0.15  SphereRadiusUnits=m  EllipsoidRadii=[1 1 1]  EllipsoidRadiiUnits=m  ExtrusionCrossSection=[1 1; -1 1; -1 -1; 1 -1]  ExtrusionCrossSectionUnits=m  ExtrusionLength=1  ExtrusionLengthUnits=m  PolygonNumSides=3  PolygonOuterRadius=1  PolygonOuterRadiusUnits=m  ExtGeomFileType=STL  ExtGeomFileUnits=m  RevolutionCrossSection=[1 1; 1 -1; 2 -1; 2 1]  RevolutionCrossSectionUnits=m  RevolutionExtent=Full  RevolutionAngle=180  RevolutionAngleUnits=deg  BlockFunction=simmechanics.library.body_elements.solid
  World Frame{,1..5} (6 alike) : sm_lib/Frames and Transforms/World Frame  BlockFunction=simmechanics.library.frames_transforms.world_frame
  World to Roll Frame : sm_lib/Frames and Transforms/Rigid Transform  TranslationMethod=None  TranslationLengthUnit=m  TranslationStandardAxis=+Z  TranslationStandardOffset=0  TranslationCartesianOffset=[0 0 0]  TranslationROffset=0  TranslationROffsetUnits=m  TranslationZOffset=0  TranslationZOffsetUnits=m  TranslationThetaOffset=0  TranslationThetaOffsetUnits=deg  RotationMethod=AlignedAxes  RotationAngleUnits=deg  RotationStandardAxis=+Z  RotationAngle=0.0  RotationArbitraryAxis=[0 0 1]  FollAlignAxisA=+Z  BaseAlignAxisA=+X  FollAlignAxisB=+Y  BaseAlignAxisB=+Y  RotationMatrix=[1 0 0; 0 1 0; 0 0 1]  BlockFunction=simmechanics.library.frames_transforms.rigid_transform
  Xb velocity comparison : Scope  NumInputPorts=2
      settings: YMin=0.95~0.95  YMax=1.05~1.05  SampleInput=on
  Yaw Joint : sm_lib/Joints/Revolute Joint  Commented=on  SenseConstraintForce=off  SenseConstraintForceX=off  SenseConstraintForceY=off  SenseConstraintForceZ=off  SenseConstraintTorque=off  SenseConstraintTorqueX=off  SenseConstraintTorqueY=off  SenseConstraintTorqueZ=off  SenseTotalForce=off  SenseTotalForceX=off  SenseTotalForceY=off  SenseTotalForceZ=off  SenseTotalTorque=off  SenseTotalTorqueX=off  SenseTotalTorqueY=off  SenseTotalTorqueZ=off  CompositeWrenchDir=FollowerOnBase  CompositeWrenchFrame=BaseFrame  EquilibriumPosition=0  EquilibriumPositionUnits=deg  SpringStiffness=0  SpringStiffnessUnits=N*m/deg  DampingCoefficient=0  DampingCoefficientUnits=N*m/(deg/s)  TorqueActuationMode=InputTorque  MotionActuationMode=ComputedMotion  SensePosition=on  SenseVelocity=on  SenseAcceleration=on  SenseTorqueForce=off  PositionTargetSpecify=on  PositionTargetPriority=High  PositionTargetValue=0  PositionTargetValueUnits=deg  VelocityTargetSpecify=off  VelocityTargetPriority=High  VelocityTargetValue=0  VelocityTargetValueUnits=deg/s  BlockFunction=simmechanics.library.joints.revolute_joint
  world to yawed : Subsystem
  world to yawed1 : Subsystem
  world to yawed2 : Subsystem
  world to yawed3 : Subsystem
  world to yawed4 : Subsystem
  world to yawed5 : Subsystem
  world to yawed6 : Subsystem
  wires:
  Sine Wave/1 -> [Z_GRF], Simulink-PS Converter4/1
  Constant1/1 -> Simulink-PS Converter1/1
  Constant2/1 -> Simulink-PS Converter/1
  PS-Simulink Converter5/1 -> Mux4/3
  PS-Simulink Converter4/1 -> Mux4/2
  PS-Simulink Converter3/1 -> Sum2/2
  PS-Simulink Converter2/1 -> Gain5/1
  PS-Simulink Converter1/1 -> Gain4/1
  PS-Simulink Converter/1 -> Sum1/2
  Mux74/1 -> world to yawed1/4(ddx_w), [RightHipComAccelerationWorld]
  [RightHipComAccelerationWorld] -> Gain1/1
  [LeftHipComAccelerationWorld] -> Gain/1
  [TorsoComAccelerationWorld] -> Gain2/1
  Gain/1 -> Sum/2
  Gain2/1 -> Sum/3
  Gain1/1 -> Sum/1
  Sum/1 -> Gain3/1
  Demux/1 -> Mux6/1
  Demux/2 -> Mux7/1
  Demux/3 -> Mux8/1
  Mux4/1 -> [RightHipAngularState], Demux1/1
  Gain4/1 -> Mux3/2
  Gain5/1 -> Mux3/3
  Sum1/1 -> Mux3/1
  Constant3/1 -> Sum1/1
  Sum2/1 -> Mux4/1
  Constant4/1 -> Sum2/1
  Demux1/1 -> Right Hip Angular Positions / Velocities / Accelerations/1
  Demux1/2 -> Right Hip Angular Positions / Velocities / Accelerations/2
  Demux1/3 -> Right Hip Angular Positions / Velocities / Accelerations/3
  Mux3/1 -> Demux2/1, [LeftHipAngularState]
  Demux2/3 -> Left Hip Angular Positions / Velocities / Accelerations/3
  Demux2/2 -> Left Hip Angular Positions / Velocities / Accelerations/2
  Demux2/1 -> Left Hip Angular Positions / Velocities / Accelerations/1
  Mux6/1 -> System COM Acceleration World Frame/1
  Mux7/1 -> System COM Acceleration World Frame/2
  Mux8/1 -> System COM Acceleration World Frame/3
  Demux3/1 -> Mux6/2
  Demux3/2 -> Mux7/2
  Demux3/3 -> Mux8/2
  [LeftHipAngularState] -> Selector2/1, Selector/1
  [RightHipAngularState] -> Selector3/1, Selector1/1
  Selector1/1 -> Compute COM Translational Acceleration (IMU uses non-rotating measurement frame)/9(right_hip_roll)
  Selector/1 -> Compute COM Translational Acceleration (IMU uses non-rotating measurement frame)/10(left_hip_roll)
  Selector2/1 -> Mux9/2
  Mux9/1 -> Compute COM Translational Acceleration (IMU uses non-rotating measurement frame)/8(hip_roll_accelerations)
  Selector3/1 -> Mux9/1
  [ImuAccelerationBody] -> Compute COM Translational Acceleration (IMU uses non-rotating measurement frame)/2(imu_translational_accelerations_body)
  [TorsoAngularAcceleration] -> Compute COM Translational Acceleration (IMU uses non-rotating measurement frame)/1(torso_angular_accelerations)
  [RollStateWorld] -> Selector4/1
  Mux5/1 -> Torso COM Acceleration World Frame/1
  Mux21/1 -> Torso COM Acceleration World Frame/2
  Mux22/1 -> Torso COM Acceleration World Frame/3
  [TorsoComAccelerationWorld] -> Demux10/1
  Demux10/1 -> Mux5/1
  Demux10/2 -> Mux21/1
  Demux10/3 -> Mux22/1
  Demux9/1 -> Mux5/2
  Demux9/2 -> Mux21/2
  Demux9/3 -> Mux22/2
  Demux11/1 -> Mux25/2
  Demux11/2 -> Mux23/2
  Demux11/3 -> Mux24/2
  Mux25/1 -> Torso COM Acceleration Relative to IMU/1
  Mux23/1 -> Torso COM Acceleration Relative to IMU/2
  Mux24/1 -> Torso COM Acceleration Relative to IMU/3
  PS-Simulink Converter6/1 -> Mux26/1
  PS-Simulink Converter7/1 -> Mux26/2
  PS-Simulink Converter8/1 -> Mux26/3
  Demux12/1 -> Mux25/1
  Demux12/2 -> Mux23/1
  Demux12/3 -> Mux24/1
  PS-Simulink Converter12/1 -> Mux27/1
  PS-Simulink Converter28/1 -> Mux27/2
  PS-Simulink Converter29/1 -> Mux27/3
  Demux13/1 -> Mux30/2  "calculation"
  Demux13/2 -> Mux28/2
  Demux13/3 -> Mux29/2
  Mux30/1 -> Torso COM Velocity Relative to IMU/1
  Mux28/1 -> Torso COM Velocity Relative to IMU/2
  Mux29/1 -> Torso COM Velocity Relative to IMU/3
  Demux14/1 -> Mux30/1  "measurement"
  Demux14/2 -> Mux28/1
  Demux14/3 -> Mux29/1
  PS-Simulink Converter40/1 -> Mux38/1
  PS-Simulink Converter41/1 -> Mux38/2
  PS-Simulink Converter42/1 -> Mux38/3
  Constant5/1 -> Simulink-PS Converter2/1
  PS-Simulink Converter44/1 -> Mux42/2
  PS-Simulink Converter43/1 -> Mux42/3
  PS-Simulink Converter45/1 -> Mux42/1
  PS-Simulink Converter32/1 -> Mux32/2
  PS-Simulink Converter31/1 -> Mux32/1
  PS-Simulink Converter33/1 -> Mux32/3
  PS-Simulink Converter34/1 -> Mux36/1
  PS-Simulink Converter35/1 -> Mux36/2
  PS-Simulink Converter36/1 -> Mux36/3
  Mux44/1 -> Imu to Torso COM yawed/1
  Mux37/1 -> Imu to Torso COM yawed/2
  Mux43/1 -> Imu to Torso COM yawed/3
  Demux18/1 -> Mux44/1
  Demux18/2 -> Mux37/1
  Demux18/3 -> Mux43/1
  [TorsoComRelativePosition] -> Demux19/1
  Demux19/1 -> Mux44/2
  Demux19/2 -> Mux37/2
  Demux19/3 -> Mux43/2
  Selector8/1 -> Mux45/1
  Selector9/1 -> Mux45/2
  Mux45/1 -> "Torso Position, Velocity, Acceleration"/1, [TorsoAngularPosition]
  [RollStateWorld] -> Selector8/1
  [PitchStateWorld] -> Selector9/1
  Selector10/1 -> Mux46/1
  Selector11/1 -> Mux46/2
  Mux46/1 -> "Torso Position, Velocity, Acceleration"/2, [TorsoAngularVelocity]
  [RollStateWorld] -> Selector10/1
  [PitchStateWorld] -> Selector11/1
  Selector12/1 -> Mux47/1
  Selector13/1 -> Mux47/2
  Mux47/1 -> "Torso Position, Velocity, Acceleration"/3, [TorsoAngularAcceleration]
  [RollStateWorld] -> Selector12/1
  [PitchStateWorld] -> Selector13/1
  Demux16/1 -> Mux41/2
  Demux16/2 -> Mux39/2
  Demux16/3 -> Mux40/2
  Mux41/1 -> IMU Acceleration Yawed/1
  Mux39/1 -> IMU Acceleration Yawed/2
  Mux40/1 -> IMU Acceleration Yawed/3
  [ImuAccelerationWorld] -> Demux17/1
  Demux17/1 -> Mux41/1
  Demux17/2 -> Mux39/1
  Demux17/3 -> Mux40/1
  PS-Simulink Converter37/1 -> Mux48/2
  PS-Simulink Converter39/1 -> Mux48/1
  PS-Simulink Converter38/1 -> Mux48/3
  Mux48/1 -> [ImuAccelerationBody]
  PS-Simulink Converter46/1 -> Mux49/2
  PS-Simulink Converter48/1 -> Mux49/1
  PS-Simulink Converter47/1 -> Mux49/3
  PS-Simulink Converter49/1 -> Mux50/2
  PS-Simulink Converter51/1 -> Mux50/1
  PS-Simulink Converter50/1 -> Mux50/3
  Mux50/1 -> [ImuPositionBody]
  Mux49/1 -> [ImuVelocityBody]
  [ImuPositionBody] -> Derivative3/1
  [ImuVelocityBody] -> Mux53/2
  Mux53/1 -> Xb velocity comparison/1
  Mux51/1 -> Xb velocity comparison/2
  Derivative3/1 -> Derivative5/1, Mux53/1
  Derivative5/1 -> Mux51/1
  [ImuAccelerationBody] -> Mux51/2
  Demux20/1 -> Mux56/2
  Demux20/2 -> Mux54/2
  Demux20/3 -> Mux55/2
  Mux56/1 -> IMU Velocity Yawed/1
  Mux54/1 -> IMU Velocity Yawed/2
  Mux55/1 -> IMU Velocity Yawed/3
  [ImuVelocityWorld] -> Demux21/1
  Demux21/1 -> Mux56/1
  Demux21/2 -> Mux54/1
  Demux21/3 -> Mux55/1
  Selector4/1 -> Compute COM Translational Acceleration (IMU uses non-rotating measurement frame)/3(torso_roll)
  [PitchStateWorld] -> Selector5/1
  Selector5/1 -> Compute COM Translational Acceleration (IMU uses non-rotating measurement frame)/4(torso_pitch)
  PS-Simulink Converter55/1 -> Mux11/2
  PS-Simulink Converter57/1 -> Mux11/1
  PS-Simulink Converter56/1 -> Mux11/3
  Mux11/1 -> [PelvisToRHipAcceleration]
  PS-Simulink Converter58/1 -> Mux12/2
  PS-Simulink Converter60/1 -> Mux12/1
  PS-Simulink Converter59/1 -> Mux12/3
  PS-Simulink Converter61/1 -> Mux57/2
  PS-Simulink Converter63/1 -> Mux57/1
  PS-Simulink Converter62/1 -> Mux57/3
  Mux57/1 -> [PelvisToRHip]
  Mux12/1 -> [PelvisToRHipVelocity]
  Demux22/1 -> Mux60/2
  Demux22/2 -> Mux58/2
  Demux22/3 -> Mux59/2
  Mux60/1 -> RHip  body frame/1
  Mux58/1 -> RHip  body frame/2
  Mux59/1 -> RHip  body frame/3
  [PelvisToRHipAcceleration] -> Demux23/1
  Demux23/1 -> Mux60/1
  Demux23/2 -> Mux58/1
  Demux23/3 -> Mux59/1
  PS-Simulink Converter64/1 -> Mux61/2
  PS-Simulink Converter66/1 -> Mux61/1
  PS-Simulink Converter65/1 -> Mux61/3
  Mux61/1 -> [PelvisToLHipAcceleration]
  PS-Simulink Converter67/1 -> Mux62/2
  PS-Simulink Converter69/1 -> Mux62/1
  PS-Simulink Converter68/1 -> Mux62/3
  PS-Simulink Converter70/1 -> Mux63/2
  PS-Simulink Converter72/1 -> Mux63/1
  PS-Simulink Converter71/1 -> Mux63/3
  Mux63/1 -> [PelvisToLHip]
  Mux62/1 -> [PelvisToLHipVelocity]
  Demux24/1 -> Mux66/2
  Demux24/2 -> Mux64/2
  Demux24/3 -> Mux65/2
  Mux66/1 -> LHip  body frame/1
  Mux64/1 -> LHip  body frame/2
  Mux65/1 -> LHip  body frame/3
  [PelvisToLHipAcceleration] -> Demux25/1
  Demux25/1 -> Mux66/1
  Demux25/2 -> Mux64/1
  Demux25/3 -> Mux65/1
  Demux4/1 -> Mux15/2
  Demux4/2 -> Mux13/2
  Demux4/3 -> Mux14/2
  Mux15/1 -> R Hip Yawed/1
  Mux13/1 -> R Hip Yawed/2
  Mux14/1 -> R Hip Yawed/3
  [RightHipComAcceleration] -> Demux5/1
  Demux5/1 -> Mux15/1
  Demux5/2 -> Mux13/1
  Demux5/3 -> Mux14/1
  Demux6/1 -> Mux18/2
  Demux6/2 -> Mux16/2
  Demux6/3 -> Mux17/2
  Mux18/1 -> L Hip Yawed/1
  Mux16/1 -> L Hip Yawed/2
  Mux17/1 -> L Hip Yawed/3
  [LeftHipComAcceleration] -> Demux7/1
  Demux7/1 -> Mux18/1
  Demux7/2 -> Mux16/1
  Demux7/3 -> Mux17/1
  [RollStateWorld] -> Selector6/1
  Selector6/1 -> PositionUsingRobotGeometry/1(roll)
  [PitchStateWorld] -> Selector7/1
  Selector7/1 -> PositionUsingRobotGeometry/2(pitch)
  Selector33/1 -> PositionUsingRobotGeometry/3(yaw)
  [LeftHipAngularState] -> Selector14/1
  [RightHipAngularState] -> Selector15/1
  Selector14/1 -> PositionUsingRobotGeometry/4(left_leg_lateral_angle)
  Selector15/1 -> PositionUsingRobotGeometry/5(right_leg_lateral_angle)
  PositionUsingRobotGeometry/1(com_pelvis) -> Kalman Filtering/2("COM from Right Foot [body, yawed, global]"), Kalman Filtering/1("COM from Left Foot [body, yawed, global]"), Selector16/1
  Mux31/1 -> COM from pelvis/1
  Mux19/1 -> COM from pelvis/2
  Mux20/1 -> COM from pelvis/3
  Demux8/1 -> Mux31/1
  Demux8/2 -> Mux19/1
  Demux8/3 -> Mux20/1
  Demux15/1 -> Mux31/2
  Demux15/2 -> Mux19/2
  Demux15/3 -> Mux20/2
  PS-Simulink Converter22/1 -> Mux33/2
  PS-Simulink Converter24/1 -> Mux33/1
  PS-Simulink Converter23/1 -> Mux33/3
  PS-Simulink Converter25/1 -> Mux34/2
  PS-Simulink Converter26/1 -> Mux34/1
  PS-Simulink Converter27/1 -> Mux34/3
  PS-Simulink Converter30/1 -> Mux35/2
  PS-Simulink Converter74/1 -> Mux35/1
  PS-Simulink Converter73/1 -> Mux35/3
  [RightHipComPositionWorld] -> Gain7/1
  [LeftHipComPositionWorld] -> Gain6/1
  [TorsoComPositionWorld] -> Gain8/1
  Gain6/1 -> Sum3/2
  Gain8/1 -> Sum3/3
  Gain7/1 -> Sum3/1
  Sum3/1 -> Gain9/1
  [LeftHipAngularState] -> Right and Left Hip Angles/2
  [RightHipAngularState] -> Right and Left Hip Angles/1
  Derivative/1 -> Mux67/2, Derivative4/1
  Derivative1/1 -> Mux68/2, Derivative6/1
  Derivative4/1 -> Mux67/3
  Mux67/1 -> [RollStateWorld]
  Derivative6/1 -> Mux68/3
  Mux68/1 -> [PitchStateWorld]
  Mux69/1 -> Torso Roll Pitch Comparison Position/1
  Mux70/1 -> Torso Roll Pitch Comparison Position/2
  Selector17/1 -> Mux69/1
  Selector18/1 -> Mux70/1
  [RollStateWorld] -> Selector19/1
  Selector19/1 -> Mux69/2
  Selector20/1 -> Mux70/2
  [PitchStateWorld] -> Selector20/1
  PositionUsingRobotGeometry/2(dcom_pelvis) -> Selector21/1
  Selector16/1 -> Derivative8/1, Demux8/1
  Gain9/1 -> [SystemComPositionWorld], Demux15/1
  [TorsoComRelativeAcceleration] -> Demux12/1
  [TorsoComRelativeVelocity] -> Demux14/1
  PS-Simulink Converter75/1 -> Rotation To Euler Angles/1(R)
  Rotation To Euler Angles/1(roll) -> Transform Roll Pitch Yaw/1, Derivative/1, Mux67/1
  Rotation To Euler Angles/2(pitch) -> Transform Roll Pitch Yaw/2, Mux68/1, Derivative1/1
  Mux36/1 -> Selector25/1, Selector18/1
  Mux32/1 -> Selector22/1, Selector17/1
  Mux71/1 -> Torso Roll Pitch Comparison Velocity/1
  Mux72/1 -> Torso Roll Pitch Comparison Velocity/2
  Selector22/1 -> Mux71/1
  Selector25/1 -> Mux72/1
  [RollStateWorld] -> Selector24/1
  Selector24/1 -> Mux71/2
  Selector23/1 -> Mux72/2
  [PitchStateWorld] -> Selector23/1
  Derivative2/1 -> Derivative7/1, Mux73/2
  Derivative7/1 -> Mux73/3
  Mux73/1 -> [YawStateWorld]
  Rotation To Euler Angles/3(yaw) -> Transform Roll Pitch Yaw/3, Mux73/1, Derivative2/1
  [YawStateWorld] -> Selector26/1
  Selector26/1 -> Compute COM Translational Acceleration (IMU uses non-rotating measurement frame)/5(torso_yaw)
  Mux34/1 -> Rotate to from World to Yawed Frame3/1(world)
  [YawStateWorld] -> Selector30/1
  Selector30/1 -> Rotate to from World to Yawed Frame3/2(yaw)
  Rotate to from World to Yawed Frame3/1(yawed) -> [RightHipComPosition]
  Mux38/1 -> world to yawed/2(x_w)
  [YawStateWorld] -> world to yawed/1(yaw_dyaw_ddyaw)
  Mux27/1 -> world to yawed/3(dx_w)
  Mux26/1 -> world to yawed/4(ddx_w)
  world to yawed/1(x_y) -> [TorsoComRelativePosition]
  world to yawed/2(dx_y) -> [TorsoComRelativeVelocity]
  world to yawed/3(ddx_y) -> [TorsoComRelativeAcceleration]
  PS-Simulink Converter82/1 -> Mux74/1
  PS-Simulink Converter83/1 -> Mux74/2
  PS-Simulink Converter84/1 -> Mux74/3
  PS-Simulink Converter76/1 -> Mux75/1
  PS-Simulink Converter77/1 -> Mux75/2
  PS-Simulink Converter78/1 -> Mux75/3
  PS-Simulink Converter79/1 -> Mux76/1
  PS-Simulink Converter80/1 -> Mux76/2
  PS-Simulink Converter81/1 -> Mux76/3
  [YawStateWorld] -> world to yawed1/1(yaw_dyaw_ddyaw)
  Mux75/1 -> world to yawed1/3(dx_w)
  Mux76/1 -> world to yawed1/2(x_w), [RightHipComPositionWorld]
  PS-Simulink Converter87/1 -> Mux78/1
  PS-Simulink Converter9/1 -> Mux2/2
  PS-Simulink Converter11/1 -> Mux2/1
  PS-Simulink Converter10/1 -> Mux2/3
  PS-Simulink Converter16/1 -> Mux77/2
  PS-Simulink Converter18/1 -> Mux77/1
  PS-Simulink Converter17/1 -> Mux77/3
  PS-Simulink Converter85/1 -> Mux78/2
  PS-Simulink Converter86/1 -> Mux78/3
  Mux35/1 -> Rotate to from World to Yawed Frame1/1(world)
  [YawStateWorld] -> Selector27/1
  Selector27/1 -> Rotate to from World to Yawed Frame1/2(yaw)
  Rotate to from World to Yawed Frame1/1(yawed) -> [TorsoComPosition]
  Mux78/1 -> [TorsoComPositionWorld], world to yawed2/2(x_w)
  [YawStateWorld] -> world to yawed2/1(yaw_dyaw_ddyaw)
  Mux77/1 -> world to yawed2/3(dx_w)
  Mux33/1 -> Rotate to from World to Yawed Frame2/1(world)
  [YawStateWorld] -> Selector28/1
  Selector28/1 -> Rotate to from World to Yawed Frame2/2(yaw)
  Rotate to from World to Yawed Frame2/1(yawed) -> [LeftHipComPosition]
  PS-Simulink Converter92/1 -> Mux80/1
  PS-Simulink Converter93/1 -> Mux1/2
  PS-Simulink Converter14/1 -> Mux1/1
  PS-Simulink Converter13/1 -> Mux1/3
  PS-Simulink Converter15/1 -> Mux79/2
  PS-Simulink Converter89/1 -> Mux79/1
  PS-Simulink Converter88/1 -> Mux79/3
  PS-Simulink Converter90/1 -> Mux80/2
  PS-Simulink Converter91/1 -> Mux80/3
  [YawStateWorld] -> world to yawed3/1(yaw_dyaw_ddyaw)
  Mux79/1 -> world to yawed3/3(dx_w)
  Mux80/1 -> world to yawed3/2(x_w), [LeftHipComPositionWorld]
  Mux1/1 -> world to yawed3/4(ddx_w), [LeftHipComAccelerationWorld]
  [YawStateWorld] -> world to yawed4/1(yaw_dyaw_ddyaw)
  PS-Simulink Converter94/1 -> Mux10/1
  PS-Simulink Converter95/1 -> Mux10/2
  PS-Simulink Converter96/1 -> Mux10/3
  PS-Simulink Converter19/1 -> Mux52/1
  PS-Simulink Converter20/1 -> Mux52/2
  PS-Simulink Converter21/1 -> Mux52/3
  PS-Simulink Converter52/1 -> Mux81/1
  PS-Simulink Converter53/1 -> Mux81/2
  PS-Simulink Converter54/1 -> Mux81/3
  Mux81/1 -> world to yawed4/2(x_w)
  Mux52/1 -> world to yawed4/3(dx_w)
  Mux10/1 -> world to yawed4/4(ddx_w)
  Sine Wave1/1 -> [Y_GRF], Simulink-PS Converter3/1
  world to yawed4/3(ddx_y) -> [ImuAccelerationWorld]
  Demux26/1 -> Mux84/2
  Demux26/2 -> Mux82/2
  Demux26/3 -> Mux83/2
  Mux84/1 -> Pelvis Acceleration from IMU Yawed/1
  Mux82/1 -> Pelvis Acceleration from IMU Yawed/2
  Mux83/1 -> Pelvis Acceleration from IMU Yawed/3
  [PelvisAccelerationFromImu] -> Demux27/1
  Demux27/1 -> Mux84/1
  Demux27/2 -> Mux82/1
  Demux27/3 -> Mux83/1
  PS-Simulink Converter103/1 -> Mux85/1
  PS-Simulink Converter104/1 -> Mux85/2
  PS-Simulink Converter105/1 -> Mux85/3
  PS-Simulink Converter97/1 -> Mux86/1
  PS-Simulink Converter98/1 -> Mux86/2
  PS-Simulink Converter99/1 -> Mux86/3
  PS-Simulink Converter100/1 -> Mux87/1
  PS-Simulink Converter101/1 -> Mux87/2
  PS-Simulink Converter102/1 -> Mux87/3
  Mux87/1 -> world to yawed5/2(x_w)
  [YawStateWorld] -> world to yawed5/1(yaw_dyaw_ddyaw)
  Mux86/1 -> world to yawed5/3(dx_w)
  Mux85/1 -> world to yawed5/4(ddx_w)
  world to yawed5/3(ddx_y) -> [PelvisAccelerationFromImu]
  Demux28/1 -> Mux90/2
  Demux28/2 -> Mux88/2
  Demux28/3 -> Mux89/2
  Mux90/1 -> Pelvis Acceleration from Ground Yawed/1
  Mux88/1 -> Pelvis Acceleration from Ground Yawed/2
  Mux89/1 -> Pelvis Acceleration from Ground Yawed/3
  [PelvisAccelerationFromGround] -> Demux29/1
  Demux29/1 -> Mux90/1
  Demux29/2 -> Mux88/1
  Demux29/3 -> Mux89/1
  PS-Simulink Converter109/1 -> Mux91/1
  PS-Simulink Converter110/1 -> Mux91/2
  PS-Simulink Converter111/1 -> Mux91/3
  PS-Simulink Converter112/1 -> Mux92/1
  PS-Simulink Converter113/1 -> Mux92/2
  PS-Simulink Converter114/1 -> Mux92/3
  PS-Simulink Converter107/1 -> Mux93/2
  PS-Simulink Converter108/1 -> Mux93/3
  Mux93/1 -> world to yawed6/2(x_w)
  [YawStateWorld] -> world to yawed6/1(yaw_dyaw_ddyaw)
  Mux92/1 -> world to yawed6/3(dx_w)
  Mux91/1 -> world to yawed6/4(ddx_w), [PelvisAccelerationWorld]
  world to yawed6/3(ddx_y) -> [PelvisAccelerationFromGround]
  PS-Simulink Converter106/1 -> Mux93/1
  [YawStateWorld] -> Selector29/1
  [YawStateWorld] -> Selector31/1
  [YawStateWorld] -> Selector32/1
  Selector32/1 -> Mux45/3
  Selector31/1 -> Mux46/3
  Selector29/1 -> Mux47/3
  [YawStateWorld] -> Selector33/1
  world to yawed2/2(dx_y) -> [TorsoComVelocity]
  Demux30/1 -> Mux96/2
  Demux30/2 -> Mux94/2
  Demux30/3 -> Mux95/2
  Mux96/1 -> Torso Velocity Yawed/1
  Mux94/1 -> Torso Velocity Yawed/2
  Mux95/1 -> Torso Velocity Yawed/3
  [TorsoComVelocity] -> Demux31/1
  Demux31/1 -> Mux96/1
  Demux31/2 -> Mux94/1
  Demux31/3 -> Mux95/1
  world to yawed4/2(dx_y) -> [ImuVelocityWorld]
  Constant/1 -> Kalman Filtering/3(GRFx [N])
  [Z_GRF] -> Kalman Filtering/5(GRFz [N])
  [Y_GRF] -> Kalman Filtering/4(GRFy [N])
  Constant6/1 -> Kalman Filtering/7(Left Vertical GRF [N])
  Constant7/1 -> Kalman Filtering/8("Initial [x, dx, ddx] [m, m/s, m/s^2]")
  Constant8/1 -> Kalman Filtering/9("Initial [y, dy, ddy] [m, m/s, m/s^2]")
  Constant9/1 -> Kalman Filtering/10("Initial [z, dz, ddz] [m m/s m/s^2]")
  Gain3/1 -> Demux/1
  [COM_acceleration_yawed] -> Kalman Filtering/11(COM XYZ Acceleration [m/s^2] x3)
  Mux99/1 -> Kalman Filter/1
  Mux97/1 -> Kalman Filter/2
  Mux98/1 -> Kalman Filter/3
  Selector34/1 -> Mux99/1
  Selector35/1 -> Mux97/1
  Selector36/1 -> Mux98/1
  Demux33/1 -> Mux99/2
  Demux33/2 -> Mux97/2
  Demux33/3 -> Mux98/2
  Kalman Filtering/1("[x, dx, ddx] [m/s, m/s^2]") -> Selector34/1
  Kalman Filtering/2("[y, dy, ddy] [m/s, m/s^2]") -> Selector35/1
  Kalman Filtering/3("[z, dz, ddz] [m, m/s, m/s^2]") -> Selector36/1
  Constant10/1 -> Kalman Filtering/Enable
  Constant11/1 -> Kalman Filtering/6(Right Vertical GRF [N])
  Constant12/1 -> Kalman Filtering/12(Entering Stance [1/0])
  Derivative8/1 -> Derivative9/1
  [COM_acceleration_yawed] -> Demux33/1
  Mux105/1 -> Pelvis to COM Accleration Yawed/1
  Mux103/1 -> Pelvis to COM Accleration Yawed/2
  Mux104/1 -> Pelvis to COM Accleration Yawed/3
  Derivative9/1 -> Demux34/1
  Demux34/1 -> Mux105/1
  Demux34/2 -> Mux103/1
  Demux34/3 -> Mux104/1
  ? -> Demux35/1
  Demux35/1 -> Mux105/2
  Demux35/2 -> Mux103/2
  Demux35/3 -> Mux104/2
  Derivative10/1 -> Derivative11/1
  Mux102/1 -> Torso COM Yawed Accel/1
  Mux100/1 -> Torso COM Yawed Accel/2
  Mux101/1 -> Torso COM Yawed Accel/3
  Derivative11/1 -> Demux32/1
  Demux32/1 -> Mux102/1
  Demux32/2 -> Mux100/1
  Demux32/3 -> Mux101/1
  Mux2/1 -> [TorsoComAccelerationWorld], world to yawed2/4(ddx_w)
  Demux36/1 -> Mux102/2
  Demux36/2 -> Mux100/2
  Demux36/3 -> Mux101/2
  world to yawed2/1(x_y) -> Derivative10/1
  Compute COM Translational Acceleration (IMU uses non-rotating measurement frame)/1(com_acceleration_world) -> Demux3/1
  Compute COM Translational Acceleration (IMU uses non-rotating measurement frame)/2(torso_com_acceleration_world) -> Demux9/1
  Mux108/1 -> Pelvis Acceleration World Frame/1
  Mux106/1 -> Pelvis Acceleration World Frame/2
  Mux107/1 -> Pelvis Acceleration World Frame/3
  [PelvisAccelerationWorld] -> Demux37/1
  Demux37/1 -> Mux108/1
  Demux37/2 -> Mux106/1
  Demux37/3 -> Mux107/1
  Demux38/1 -> Mux108/2
  Demux38/2 -> Mux106/2
  Demux38/3 -> Mux107/2
  Compute COM Translational Acceleration (IMU uses non-rotating measurement frame)/3(pelvis_acceleration_world) -> Demux38/1
  Mux111/1 -> Right Hip Acceleration World Frame/1
  Mux109/1 -> Right Hip Acceleration World Frame/2
  Mux110/1 -> Right Hip Acceleration World Frame/3
  [RightHipComAccelerationWorld] -> Demux39/1
  Demux39/2 -> Mux109/1
  Demux39/3 -> Mux110/1
  Demux40/1 -> Mux111/2
  Demux40/2 -> Mux109/2
  Demux40/3 -> Mux110/2
  Demux39/1 -> Mux111/1
  Compute COM Translational Acceleration (IMU uses non-rotating measurement frame)/4(right_hip_acceleration_world) -> Demux40/1
  world to yawed1/3(ddx_y) -> [RightHipComAccelerationYawed]
  Mux114/1 -> Left Hip Acceleration World Frame/1
  Mux112/1 -> Left Hip Acceleration World Frame/2
  Mux113/1 -> Left Hip Acceleration World Frame/3
  [LeftHipComAccelerationWorld] -> Demux41/1
  Demux41/2 -> Mux112/1
  Demux41/3 -> Mux113/1
  Demux42/1 -> Mux114/2
  Demux42/2 -> Mux112/2
  Demux42/3 -> Mux113/2
  Demux41/1 -> Mux114/1
  Compute COM Translational Acceleration (IMU uses non-rotating measurement frame)/5(left_hip_acceleration_world) -> Demux42/1
  [RightHipComAccelerationYawed] -> Gain11/1
  [LeftHipComAccelerationYawed] -> Gain10/1
  [TorsoComAccelerationYawed] -> Gain12/1
  Gain10/1 -> Sum4/2
  Gain12/1 -> Sum4/3
  Gain11/1 -> Sum4/1
  Sum4/1 -> Gain13/1
  [SystemComPositionWorld] -> Derivative12/1, Compute COM Translational Acceleration (IMU uses non-rotating measurement frame)/6(com_position_world)
  Derivative12/1 -> Compute COM Translational Acceleration (IMU uses non-rotating measurement frame)/7(com_velocity_world)
  Mux117/1 -> COM Acceleration Yawed Frame/1
  Mux115/1 -> COM Acceleration Yawed Frame/2
  Mux116/1 -> COM Acceleration Yawed Frame/3
  Gain13/1 -> Demux44/1
  Demux44/2 -> Mux115/1
  Demux44/3 -> Mux116/1
  Demux45/1 -> Mux117/2
  Demux45/2 -> Mux115/2
  Demux45/3 -> Mux116/2
  Demux44/1 -> Mux117/1
  Compute COM Translational Acceleration (IMU uses non-rotating measurement frame)/6(com_acceleration_yawed) -> Demux45/1
  world to yawed3/3(ddx_y) -> [LeftHipComAccelerationYawed]
  world to yawed2/3(ddx_y) -> [TorsoComAccelerationYawed]
  connections:
  World Frame/RConn1 -- Cartesian Joint/LConn1 -- Solver Configuration/RConn1 -- Mechanism Configuration/RConn1
  Right Hip Mass/RConn1 -- Pelvis to R Hip COM/LConn1 -- Pelvic Rotation to World2/RConn1
  Left Hip Mass/RConn1 -- Pelvis to L Hip COM/LConn1 -- Pelvic Rotation to World1/RConn1
  Pelvic Rotation to World/LConn1 -- World to Roll Frame/RConn1 -- Pelvis/RConn1 -- Pelvic Rotation to World3/LConn1 -- Right Hip Joint/LConn1 -- Left Hip Joint/LConn1
  PS-Simulink Converter/LConn1 -- Left Hip Joint/RConn2
  PS-Simulink Converter2/LConn1 -- Left Hip Joint/RConn4
  Left Hip Joint/RConn3 -- PS-Simulink Converter1/LConn1
  Simulink-PS Converter/RConn1 -- Left Hip Joint/LConn2
  PS-Simulink Converter3/LConn1 -- Right Hip Joint/RConn2
  Right Hip Joint/RConn3 -- PS-Simulink Converter4/LConn1
  Right Hip Joint/RConn4 -- PS-Simulink Converter5/LConn1
  Simulink-PS Converter1/RConn1 -- Right Hip Joint/LConn2
  Yaw Joint/RConn1 -- Transform Sensor/LConn1 -- Cartesian Joint/RConn1 -- Roll and Pitch Joint/LConn1
  R Hip Graphic/RConn1 -- Transform Sensor3/RConn1 -- Transform Sensor7/RConn1 -- Transform Sensor10/RConn1 -- Pelvis to R Hip COM/RConn1
  L Hip Graphic/RConn1 -- Transform Sensor8/RConn1 -- Transform Sensor2/RConn1 -- Transform Sensor9/RConn1 -- Pelvis to L Hip COM/RConn1
  Torso Graphic/RConn1 -- Transform Sensor8/LConn1 -- Transform Sensor1/RConn1 -- Transform Sensor11/RConn1 -- Transform Sensor7/LConn1 -- Transform Sensor5/RConn1 -- Pelvis to Trunk COM/RConn1
  Trunk Mass/RConn1 -- Pelvis to Trunk COM/LConn1 -- Pelvic Rotation to World/RConn1
  Pelvic Rotation to World1/LConn1 -- Left Hip Joint/RConn1
  Pelvic Rotation to World2/LConn1 -- Right Hip Joint/RConn1
  World Frame1/RConn1 -- Transform Sensor1/LConn1
  World Frame2/RConn1 -- Transform Sensor2/LConn1
  World Frame3/RConn1 -- Transform Sensor3/LConn1
  Transform Sensor4/RConn1 -- IMU/RConn1 -- Transform Sensor5/LConn1 -- Transform Sensor12/LConn1 -- Transform Sensor6/RConn1 -- Pelvis to IMU/RConn1
  Roll and Pitch Joint/RConn1 -- Transform Sensor10/LConn1 -- Transform Sensor13/RConn1 -- Transform Sensor12/RConn1 -- World to Roll Frame/LConn1 -- Transform Sensor11/LConn1 -- Transform Sensor9/LConn1 -- Transform Sensor/RConn1
  Pelvis to IMU/LConn1 -- Pelvic Rotation to World3/RConn1
  PS-Simulink Converter42/LConn1 -- Transform Sensor5/RConn4
  PS-Simulink Converter41/LConn1 -- Transform Sensor5/RConn3
  Transform Sensor5/RConn2 -- PS-Simulink Converter40/LConn1
  PS-Simulink Converter12/LConn1 -- Transform Sensor5/RConn5
  PS-Simulink Converter28/LConn1 -- Transform Sensor5/RConn6
  PS-Simulink Converter29/LConn1 -- Transform Sensor5/RConn7
  PS-Simulink Converter6/LConn1 -- Transform Sensor5/RConn8
  PS-Simulink Converter7/LConn1 -- Transform Sensor5/RConn9
  PS-Simulink Converter8/LConn1 -- Transform Sensor5/RConn10
  Simulink-PS Converter2/RConn1 -- Yaw Joint/LConn2
  PS-Simulink Converter45/LConn1 -- Yaw Joint/RConn2
  PS-Simulink Converter43/LConn1 -- Yaw Joint/RConn4
  PS-Simulink Converter44/LConn1 -- Yaw Joint/RConn3
  Roll and Pitch Joint/RConn2 -- PS-Simulink Converter31/LConn1
  Roll and Pitch Joint/RConn3 -- PS-Simulink Converter32/LConn1
  Roll and Pitch Joint/RConn4 -- PS-Simulink Converter33/LConn1
  Roll and Pitch Joint/RConn5 -- PS-Simulink Converter34/LConn1
  Roll and Pitch Joint/RConn6 -- PS-Simulink Converter35/LConn1
  Roll and Pitch Joint/RConn7 -- PS-Simulink Converter36/LConn1
  World Frame4/RConn1 -- Transform Sensor4/LConn1 -- Transform Sensor6/LConn1
  Transform Sensor6/RConn9 -- PS-Simulink Converter37/LConn1
  Transform Sensor6/RConn8 -- PS-Simulink Converter39/LConn1
  Transform Sensor6/RConn10 -- PS-Simulink Converter38/LConn1
  PS-Simulink Converter48/LConn1 -- Transform Sensor6/RConn5
  PS-Simulink Converter51/LConn1 -- Transform Sensor6/RConn2
  Transform Sensor6/RConn3 -- PS-Simulink Converter49/LConn1
  PS-Simulink Converter50/LConn1 -- Transform Sensor6/RConn4
  Transform Sensor6/RConn6 -- PS-Simulink Converter46/LConn1
  Transform Sensor6/RConn7 -- PS-Simulink Converter47/LConn1
  Transform Sensor7/RConn2 -- PS-Simulink Converter63/LConn1
  Transform Sensor7/RConn3 -- PS-Simulink Converter61/LConn1
  Transform Sensor7/RConn4 -- PS-Simulink Converter62/LConn1
  Transform Sensor7/RConn5 -- PS-Simulink Converter60/LConn1
  Transform Sensor7/RConn6 -- PS-Simulink Converter58/LConn1
  Transform Sensor7/RConn7 -- PS-Simulink Converter59/LConn1
  Transform Sensor7/RConn8 -- PS-Simulink Converter57/LConn1
  Transform Sensor7/RConn9 -- PS-Simulink Converter55/LConn1
  Transform Sensor7/RConn10 -- PS-Simulink Converter56/LConn1
  Transform Sensor8/RConn8 -- PS-Simulink Converter66/LConn1
  Transform Sensor8/RConn10 -- PS-Simulink Converter65/LConn1
  Transform Sensor8/RConn7 -- PS-Simulink Converter68/LConn1
  Transform Sensor8/RConn5 -- PS-Simulink Converter69/LConn1
  Transform Sensor8/RConn9 -- PS-Simulink Converter64/LConn1
  Transform Sensor8/RConn4 -- PS-Simulink Converter71/LConn1
  Transform Sensor8/RConn2 -- PS-Simulink Converter72/LConn1
  Transform Sensor8/RConn6 -- PS-Simulink Converter67/LConn1
  Transform Sensor8/RConn3 -- PS-Simulink Converter70/LConn1
  Simulink-PS Converter4/RConn1 -- Cartesian Joint/LConn3
  Simulink-PS Converter3/RConn1 -- Cartesian Joint/LConn2
  PS-Simulink Converter24/LConn1 -- Transform Sensor9/RConn2
  PS-Simulink Converter22/LConn1 -- Transform Sensor9/RConn3
  Transform Sensor9/RConn4 -- PS-Simulink Converter23/LConn1
  PS-Simulink Converter26/LConn1 -- Transform Sensor10/RConn2
  PS-Simulink Converter25/LConn1 -- Transform Sensor10/RConn3
  PS-Simulink Converter27/LConn1 -- Transform Sensor10/RConn4
  Transform Sensor11/RConn4 -- PS-Simulink Converter73/LConn1
  PS-Simulink Converter30/LConn1 -- Transform Sensor11/RConn3
  PS-Simulink Converter74/LConn1 -- Transform Sensor11/RConn2
  PS-Simulink Converter75/LConn1 -- Transform Sensor/RConn2
  PS-Simulink Converter79/LConn1 -- Transform Sensor3/RConn2
  Transform Sensor3/RConn3 -- PS-Simulink Converter80/LConn1
  Transform Sensor3/RConn4 -- PS-Simulink Converter81/LConn1
  Transform Sensor3/RConn5 -- PS-Simulink Converter76/LConn1
  Transform Sensor3/RConn6 -- PS-Simulink Converter77/LConn1
  Transform Sensor3/RConn7 -- PS-Simulink Converter78/LConn1
  Transform Sensor3/RConn8 -- PS-Simulink Converter82/LConn1
  Transform Sensor3/RConn9 -- PS-Simulink Converter83/LConn1
  Transform Sensor3/RConn10 -- PS-Simulink Converter84/LConn1
  PS-Simulink Converter87/LConn1 -- Transform Sensor1/RConn2
  Transform Sensor1/RConn3 -- PS-Simulink Converter85/LConn1
  Transform Sensor1/RConn4 -- PS-Simulink Converter86/LConn1
  Transform Sensor1/RConn5 -- PS-Simulink Converter18/LConn1
  Transform Sensor1/RConn6 -- PS-Simulink Converter16/LConn1
  Transform Sensor1/RConn7 -- PS-Simulink Converter17/LConn1
  Transform Sensor1/RConn8 -- PS-Simulink Converter11/LConn1
  Transform Sensor1/RConn9 -- PS-Simulink Converter9/LConn1
  Transform Sensor1/RConn10 -- PS-Simulink Converter10/LConn1
  PS-Simulink Converter92/LConn1 -- Transform Sensor2/RConn2
  Transform Sensor2/RConn3 -- PS-Simulink Converter90/LConn1
  Transform Sensor2/RConn4 -- PS-Simulink Converter91/LConn1
  Transform Sensor2/RConn5 -- PS-Simulink Converter89/LConn1
  Transform Sensor2/RConn6 -- PS-Simulink Converter15/LConn1
  Transform Sensor2/RConn7 -- PS-Simulink Converter88/LConn1
  Transform Sensor2/RConn8 -- PS-Simulink Converter14/LConn1
  PS-Simulink Converter93/LConn1 -- Transform Sensor2/RConn9
  PS-Simulink Converter13/LConn1 -- Transform Sensor2/RConn10
  PS-Simulink Converter52/LConn1 -- Transform Sensor4/RConn2
  Transform Sensor4/RConn3 -- PS-Simulink Converter53/LConn1
  Transform Sensor4/RConn4 -- PS-Simulink Converter54/LConn1
  Transform Sensor4/RConn5 -- PS-Simulink Converter19/LConn1
  Transform Sensor4/RConn6 -- PS-Simulink Converter20/LConn1
  PS-Simulink Converter21/LConn1 -- Transform Sensor4/RConn7
  PS-Simulink Converter94/LConn1 -- Transform Sensor4/RConn8
  PS-Simulink Converter95/LConn1 -- Transform Sensor4/RConn9
  PS-Simulink Converter96/LConn1 -- Transform Sensor4/RConn10
  PS-Simulink Converter105/LConn1 -- Transform Sensor12/RConn10
  PS-Simulink Converter104/LConn1 -- Transform Sensor12/RConn9
  PS-Simulink Converter103/LConn1 -- Transform Sensor12/RConn8
  PS-Simulink Converter99/LConn1 -- Transform Sensor12/RConn7
  PS-Simulink Converter98/LConn1 -- Transform Sensor12/RConn6
  PS-Simulink Converter97/LConn1 -- Transform Sensor12/RConn5
  Transform Sensor12/RConn2 -- PS-Simulink Converter100/LConn1
  PS-Simulink Converter101/LConn1 -- Transform Sensor12/RConn3
  PS-Simulink Converter102/LConn1 -- Transform Sensor12/RConn4
  PS-Simulink Converter107/LConn1 -- Transform Sensor13/RConn3
  PS-Simulink Converter112/LConn1 -- Transform Sensor13/RConn5
  PS-Simulink Converter110/LConn1 -- Transform Sensor13/RConn9
  PS-Simulink Converter109/LConn1 -- Transform Sensor13/RConn8
  PS-Simulink Converter113/LConn1 -- Transform Sensor13/RConn6
  PS-Simulink Converter114/LConn1 -- Transform Sensor13/RConn7
  PS-Simulink Converter111/LConn1 -- Transform Sensor13/RConn10
  PS-Simulink Converter108/LConn1 -- Transform Sensor13/RConn4
  Transform Sensor13/LConn1 -- World Frame5/RConn1
  PS-Simulink Converter106/LConn1 -- Transform Sensor13/RConn2
